simulink model "sampleModel200"  (Simulink 9.1)
settings: Solver=VariableStepAuto  StartTime=0.0  StopTime=10.0  RelTol=1e-3
undefined symbols (not defined in the file): DiscIntNeverNeededParam, magnitude, Newton, Raphson
libraries: simulink x23
settings Model: SuppressorTable="22 serialization::archive 11 0 6 0 0 1 8 0 0 0 0 6 0 0 1 0 22 sampleModel200/cfblk22 0 6 0 0 2 8 0 0 0 0 6 41 Simulink:DataType:WarningOverFlowDetected 0 0 0 6 0  0  0 0 0 0 8 20160608 0 0 0 15 23 17 0 1 40 SimulinkFixedPoint:util:Overflowoccurred 0 0 0  0  8 20160608 0 15 23 17 0 1"  Creator=DELL  LastModifiedBy=DELL
settings DataIOCC: SaveFormat=Dataset
settings OptimizationCC: LifeSpan=auto
settings DebuggingCC: UnderspecifiedInitializationDetection=Simplified  MergeDetectMultiDrivingBlocksExec=error  SFUnexpectedBacktrackingDiag=error  SFNoUnconditionalDefaultTransitionDiag=error  SFExecutionAtInitializationDiag=warning
settings HardwareCC: ProdBitPerPointer=64  ProdBitPerSizeT=64  ProdBitPerPtrDiffT=64  ProdLargestAtomicFloat=Float  ProdIntDivRoundTo=Zero  ProdEndianess=LittleEndian  ProdWordSize=64  ProdHWDeviceType=Intel->x86-64 (Windows64)
settings ModelReferenceCC: PropagateSignalLabelsOutOfModel=on
settings CodeAppCC: StateflowObjectComments=off
settings GRTTargetCC: TargetLangStandard=C99 (ISO)  CombineOutputUpdateFcns=on  GRTInterface=off
settings ConfigComp: CovMetricSettings=dwe  CovHtmlReporting=off  CovSaveCumulativeToWorkspaceVar=off  CovSaveSingleToWorkspaceVar=off  CovExternalEMLEnable=on

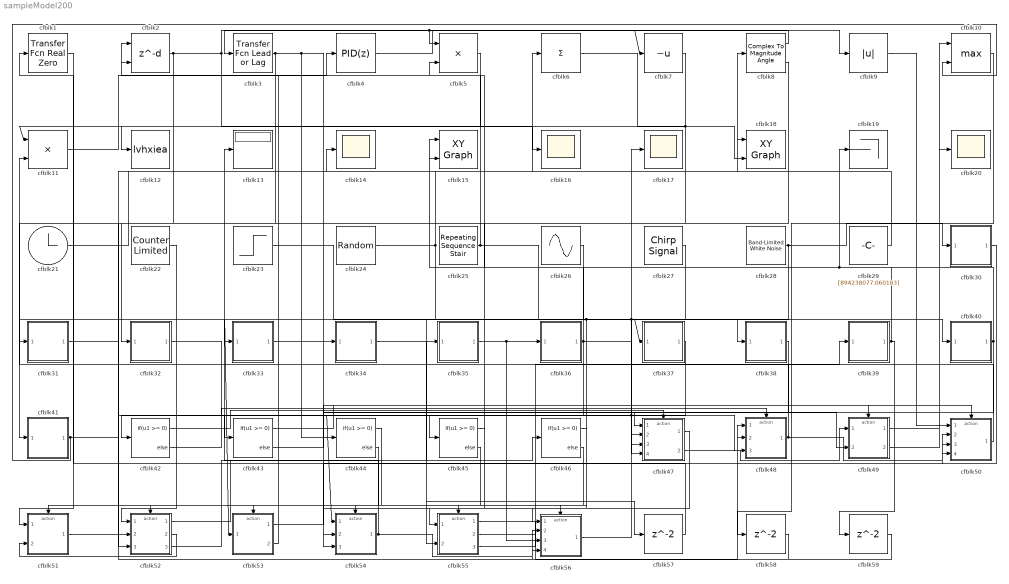
== system sampleModel200 ==
  cfblk1 : simulink/Discrete/Transfer Fcn Real Zero  ZeroZ=0.75  ICPrevInput=0.0  DoSatur=off
      settings: SourceProductName=Simulink  SourceProductBaseCode=SL
  cfblk10 : MinMax  Function=max  Inputs=2
  cfblk11 : Product
  cfblk12 : ToWorkspace  VariableName=lvhxiea  SaveFormat=Timeseries  SampleTime=-1
  cfblk13 : Display
  cfblk{14,16..17,20} (4 alike) : Scope
  cfblk15 : simulink/Sinks/XY Graph  xmin=-1  xmax=1  ymin=-1  ymax=1  st=-1
  cfblk18 : simulink/Sinks/XY Graph  xmin=-1  xmax=1  ymin=-1  ymax=1  st=-1
  cfblk19 : Terminator
  cfblk2 : Delay  DelayLengthSource=Input port  SampleTime=1
      settings: InputPortMap=u0,p1
  cfblk21 : Clock
  cfblk22 : simulink/Sources/Counter Limited  uplimit=[859.000000]  tsamp=-1
  cfblk23 : Step  Time=[38.000000]  Before=[-360941089.850897]  After=[233838912.755649]  SampleTime=0
  cfblk24 : UniformRandomNumber  Minimum=[-6461588901.663700]  Maximum=[4422499536.423707]  Seed=[95995438.000000]  SampleTime=0.1
  cfblk25 : simulink/Sources/Repeating Sequence Stair  OutValues=[-949505601.324327, -713448805.257307]  tsamp=-1  OutMin=[]  OutMax=[]  OutDataTypeStr=double  OutputDataTypeScalingMode=double  OutDataType=fixdt(0,8)  ConRadixGroup=Best Precision: Vector-wise  OutScaling=2^-12
  cfblk26 : Sin  Amplitude=[82135622.117132]  Bias=[-80870349.123243]  SampleTime=0
  cfblk27 : simulink/Sources/Chirp Signal  f1=[749318228.820739]  T=[-649807459.958066]  f2=[-242108775.631314]
  cfblk28 : simulink/Sources/Band-Limited White Noise  Cov=[6378277694.470449]  Ts=0.1  seed=[3428189316.000000]
  cfblk29 : Constant  Value=[894238077.060183]  SampleTime=1
  cfblk3 : simulink/Discrete/Transfer Fcn Lead or Lag  PoleZ=0.95  ZeroZ=0.75  ICPrevOutput=0.0  ICPrevInput=0.0  DoSatur=off
      settings: SourceProductName=Simulink  SourceProductBaseCode=SL
  cfblk30 : Subsystem
  cfblk31 : Subsystem
  cfblk32 : Subsystem
  cfblk33 : Subsystem
  cfblk34 : Subsystem
  cfblk35 : Subsystem
  cfblk36 : Subsystem
  cfblk37 : Subsystem
  cfblk38 : Subsystem
  cfblk39 : Subsystem
  cfblk4 : simulink/Continuous/PID Controller  Controller=PID  TimeDomain=Discrete-time  SampleTime=1  IntegratorMethod=Forward Euler  FilterMethod=Forward Euler  Form=Parallel  UseFilter=on  ControllerParametersSource=internal  P=1  I=1  D=0  N=100  InitialConditionSource=internal  InitialConditionForIntegrator=0  InitialConditionForFilter=0  ExternalReset=none  LimitOutput=off  UpperSaturationLimit=inf  LowerSaturationLimit=-inf  LinearizeAsGain=off  AntiWindupMode=none  Kb=1  TrackingMode=off  Kt=1  PParamMin=[]  PParamMax=[]  IParamMin=[]  IParamMax=[]  DParamMin=[]  DParamMax=[]  NParamMin=[]  NParamMax=[]  KbParamMin=[]  KbParamMax=[]  KtParamMin=[]  KtParamMax=[]  POutMin=[]  POutMax=[]  IOutMin=[]  IOutMax=[]  DOutMin=[]  DOutMax=[]  NOutMin=[]  NOutMax=[]  KbOutMin=[]  KbOutMax=[]  KtOutMin=[]  KtOutMax=[]  IntegratorOutMin=[]  IntegratorOutMax=[]  FilterOutMin=[]  FilterOutMax=[]  SumOutMin=[]  SumOutMax=[]  SumI1OutMin=[]  SumI1OutMax=[]  SumI2OutMin=[]  SumI2OutMax=[]  SumI3OutMin=[]  SumI3OutMax=[]  SumDOutMin=[]  SumDOutMax=[]  SaturationOutMin=[]  SaturationOutMax=[]  IntegratorContinuousStateAttributes=''  IntegratorStateMustResolveToSignalObject=off  IntegratorRTWStateStorageClass=Auto  FilterContinuousStateAttributes=''  FilterStateMustResolveToSignalObject=off  FilterRTWStateStorageClass=Auto  DifferentiatorICPrevScaledInput=0  DifferentiatorOutMin=[]  DifferentiatorOutMax=[]  FilterDiffOutCoefMin=[]  FilterDiffOutCoefMax=[]  SumDenOutMin=[]  SumDenOutMax=[]  SumNumOutMin=[]  SumNumOutMax=[]  ReciprocalOutMin=[]  ReciprocalOutMax=[]  DivideOutMin=[]  DivideOutMax=[]  TunerSelectOption=Transfer Function Based (PID Tuner App)
  cfblk40 : Subsystem
  cfblk41 : Subsystem
  cfblk{42..46} (5 alike) : If  IfExpression=u1 >= 0  SampleTime=1
  cfblk47 : Subsystem  TreatAsAtomicUnit=on
  cfblk48 : Subsystem  TreatAsAtomicUnit=on
  cfblk49 : Subsystem  TreatAsAtomicUnit=on
  cfblk5 : Product  Inputs=**
  cfblk50 : Subsystem  TreatAsAtomicUnit=on
  cfblk51 : Subsystem  TreatAsAtomicUnit=on
  cfblk52 : Subsystem  TreatAsAtomicUnit=on
  cfblk53 : Subsystem  TreatAsAtomicUnit=on
  cfblk54 : Subsystem  TreatAsAtomicUnit=on
  cfblk55 : Subsystem  TreatAsAtomicUnit=on
  cfblk56 : Subsystem  TreatAsAtomicUnit=on
  cfblk57 : Delay  SampleTime=1
  cfblk58 : Delay  SampleTime=1
  cfblk59 : Delay  SampleTime=1
  cfblk6 : Sum  Inputs=+
  cfblk7 : UnaryMinus
  cfblk8 : ComplexToMagnitudeAngle
  cfblk9 : Abs
  wires:
  cfblk7/1 -> cfblk11/1, cfblk55/1(cfblk1)
  cfblk48/1(cfblk2) -> cfblk11/2, cfblk50/4(cfblk12)
  cfblk21/1 -> cfblk8/1
  cfblk39/1(cfblk2) -> cfblk19/1, cfblk5/2, cfblk59/1
  cfblk23/1 -> cfblk37/1(cfblk1), cfblk47/3(cfblk15)
  cfblk9/1 -> cfblk50/1(cfblk1)
  cfblk4/1 -> cfblk9/1
  cfblk56/1(cfblk2) -> cfblk17/1
  cfblk27/1 -> cfblk53/1(cfblk1), cfblk56/1(cfblk1)
  cfblk24/1 -> cfblk6/1, cfblk38/1(cfblk1)
  cfblk8/1 -> cfblk3/1
  cfblk55/1(cfblk2) -> cfblk48/1(cfblk1)
  cfblk5/1 -> cfblk12/1
  cfblk37/1(cfblk2) -> cfblk54/1(cfblk1), cfblk47/2(cfblk14)
  cfblk49/1(cfblk2) -> cfblk10/1
  cfblk36/1(cfblk2) -> cfblk42/1, cfblk40/1(cfblk1), cfblk15/2
  cfblk49/2(cfblk10) -> cfblk20/1
  cfblk22/1 -> cfblk52/1(cfblk1)
  cfblk33/1(cfblk2) -> cfblk34/1(cfblk1)
  cfblk54/1(cfblk2) -> cfblk13/1, cfblk56/2(cfblk12)
  cfblk11/1 -> cfblk4/1
  cfblk50/1(cfblk2) -> cfblk33/1(cfblk1)
  cfblk40/1(cfblk2) -> cfblk15/1, cfblk47/1(cfblk1)
  cfblk35/1(cfblk2) -> cfblk36/1(cfblk1), cfblk56/3(cfblk13)
  cfblk29/1 -> cfblk18/1
  cfblk25/1 -> cfblk2/1, cfblk47/4(cfblk16)
  cfblk51/1(cfblk2) -> cfblk14/1
  cfblk3/1 -> cfblk44/1, cfblk49/2(cfblk9), cfblk32/1(cfblk1)
  cfblk6/1 -> cfblk18/2
  cfblk2/1 -> cfblk5/1, cfblk7/1, cfblk16/1, cfblk52/3(cfblk14)
  cfblk55/2(cfblk13) -> cfblk48/2(cfblk13)
  cfblk30/1(cfblk2) -> cfblk50/2(cfblk10)
  cfblk32/1(cfblk2) -> cfblk45/1
  cfblk8/2 -> cfblk41/1(cfblk1)
  cfblk55/3(cfblk14) -> cfblk39/1(cfblk1)
  cfblk41/1(cfblk2) -> cfblk10/2, cfblk43/1
  cfblk26/1 -> cfblk51/1(cfblk1)
  cfblk47/1(cfblk2) -> cfblk54/2(cfblk11)
  cfblk47/2(cfblk17) -> cfblk49/1(cfblk1)
  cfblk53/1(cfblk2) -> cfblk50/3(cfblk11)
  cfblk31/1(cfblk2) -> cfblk48/3(cfblk14)
  cfblk38/1(cfblk2) -> cfblk54/3(cfblk12)
  cfblk28/1 -> cfblk30/1(cfblk1), cfblk55/2(cfblk12)
  cfblk52/1(cfblk2) -> cfblk35/1(cfblk1)
  cfblk53/2(cfblk7) -> cfblk2/2
  cfblk52/2(cfblk15) -> cfblk51/2(cfblk8)
  cfblk1/1 -> cfblk31/1(cfblk1)
  cfblk52/3(cfblk16) -> cfblk46/1
  cfblk42/1 -> cfblk47/Action
  cfblk42/2 -> cfblk48/Action
  cfblk43/1 -> cfblk49/Action
  cfblk43/2 -> cfblk50/Action
  cfblk44/1 -> cfblk51/Action
  cfblk44/2 -> cfblk52/Action
  cfblk45/1 -> cfblk53/Action
  cfblk45/2 -> cfblk54/Action
  cfblk46/1 -> cfblk55/Action
  cfblk46/2 -> cfblk56/Action
  cfblk34/1(cfblk2) -> cfblk57/1
  cfblk57/1 -> cfblk1/1
  cfblk10/1 -> cfblk58/1
  cfblk58/1 -> cfblk52/2(cfblk13)
  cfblk59/1 -> cfblk56/4(cfblk14)

== system sampleModel200/cfblk30 ==
  cfblk1 : Inport
  cfblk2 : Outport
  wires:
  cfblk1/1 -> cfblk2/1

== system sampleModel200/cfblk31 ==
  cfblk1 : Inport
  cfblk2 : Outport
  wires:
  cfblk1/1 -> cfblk2/1

== system sampleModel200/cfblk32 ==
  cfblk1 : Inport
  cfblk2 : Outport
  wires:
  cfblk1/1 -> cfblk2/1

== system sampleModel200/cfblk33 ==
  cfblk1 : Inport
  cfblk2 : Outport
  wires:
  cfblk1/1 -> cfblk2/1

== system sampleModel200/cfblk34 ==
  cfblk1 : Inport
  cfblk2 : Outport
  wires:
  cfblk1/1 -> cfblk2/1

== system sampleModel200/cfblk35 ==
  cfblk1 : Inport
  cfblk2 : Outport
  wires:
  cfblk1/1 -> cfblk2/1

== system sampleModel200/cfblk36 ==
  cfblk1 : Inport
  cfblk2 : Outport
  wires:
  cfblk1/1 -> cfblk2/1

== system sampleModel200/cfblk37 ==
  cfblk1 : Inport
  cfblk2 : Outport
  wires:
  cfblk1/1 -> cfblk2/1

== system sampleModel200/cfblk38 ==
  cfblk1 : Inport
  cfblk2 : Outport
  wires:
  cfblk1/1 -> cfblk2/1

== system sampleModel200/cfblk39 ==
  cfblk1 : Inport
  cfblk2 : Outport
  wires:
  cfblk1/1 -> cfblk2/1

== system sampleModel200/cfblk40 ==
  cfblk1 : Inport
  cfblk2 : Outport
  wires:
  cfblk1/1 -> cfblk2/1

== system sampleModel200/cfblk41 ==
  cfblk1 : Inport
  cfblk2 : Outport
  wires:
  cfblk1/1 -> cfblk2/1

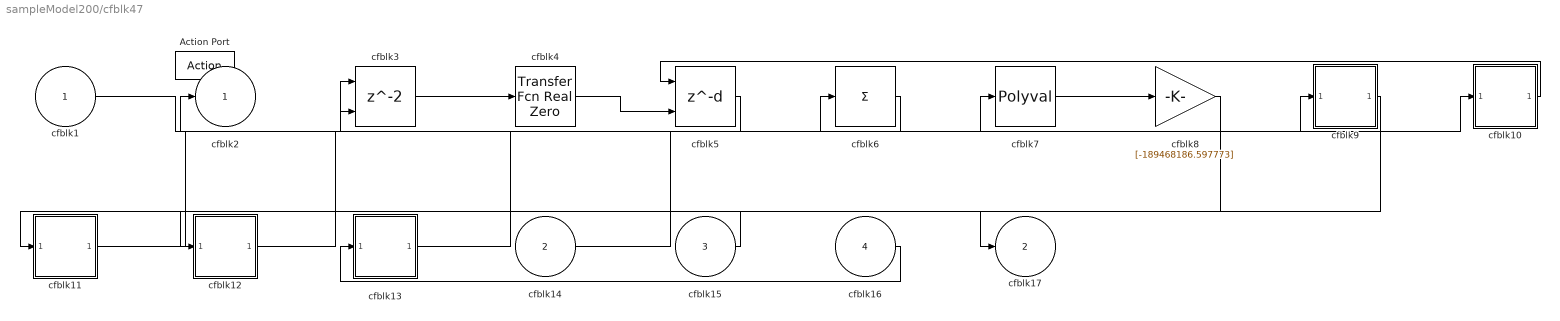
== system sampleModel200/cfblk47 ==
  cfblk1 : Inport
  cfblk14 : Inport  Port=2
  cfblk15 : Inport  Port=3
  cfblk16 : Inport  Port=4
  Action Port : ActionPort  ActionType=then
  cfblk10 : Subsystem
  cfblk11 : Subsystem
  cfblk12 : Subsystem
  cfblk13 : Subsystem
  cfblk3 : Delay  ShowEnablePort=on
      settings: InputPortMap=u0,e6
  cfblk4 : simulink/Discrete/Transfer Fcn Real Zero  ZeroZ=0.75  ICPrevInput=0.0  DoSatur=off
      settings: SourceProductName=Simulink  SourceProductBaseCode=SL
  cfblk5 : Delay  DelayLengthSource=Input port
      settings: InputPortMap=u0,p1
  cfblk6 : Sum  Inputs=+
  cfblk7 : Polyval  Coefs=[ +2.081618890e-019, -1.441693666e-014, +4.719686976e-010, -8.536869453e-006, +1.621573104e-001, -8.087801117e+001 ]
  cfblk8 : Gain  Gain=[-189468186.597773]
  cfblk9 : Subsystem
  cfblk2 : Outport
  cfblk17 : Outport  Port=2
  wires:
  cfblk7/1 -> cfblk8/1
  cfblk13/1(cfblk2) -> cfblk10/1(cfblk1)
  cfblk3/1 -> cfblk4/1
  cfblk16/1 -> cfblk13/1(cfblk1)
  cfblk14/1 -> cfblk7/1
  cfblk10/1(cfblk2) -> cfblk5/1
  cfblk11/1(cfblk2) -> cfblk3/1
  cfblk5/1 -> cfblk2/1
  cfblk4/1 -> cfblk5/2
  cfblk12/1(cfblk2) -> cfblk9/1(cfblk1)
  cfblk9/1(cfblk2) -> cfblk17/1
  cfblk15/1 -> cfblk12/1(cfblk1)
  cfblk8/1 -> cfblk11/1(cfblk1)
  cfblk6/1 -> cfblk3/2
  cfblk1/1 -> cfblk6/1

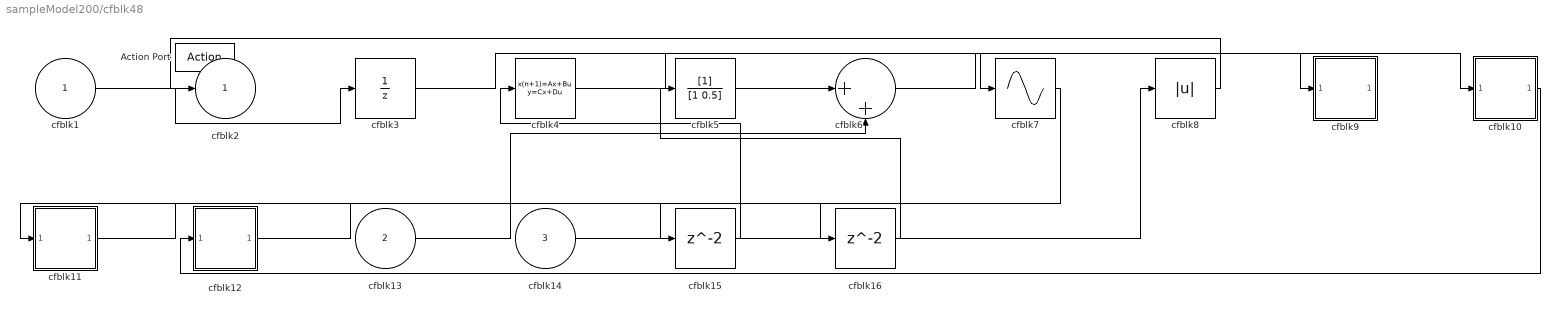
== system sampleModel200/cfblk48 ==
  cfblk1 : Inport
  cfblk13 : Inport  Port=2
  cfblk14 : Inport  Port=3
  Action Port : ActionPort  ActionType=else
  cfblk10 : Subsystem
  cfblk11 : Subsystem
  cfblk12 : Subsystem
  cfblk15 : Delay
  cfblk16 : Delay
  cfblk3 : UnitDelay  SampleTime=-1
  cfblk4 : DiscreteStateSpace  SampleTime=-1
  cfblk5 : DiscreteFilter
  cfblk6 : Sum  Inputs=|++
  cfblk7 : Sin  TimeSource=Use external signal  SampleTime=0
  cfblk8 : Abs
  cfblk9 : Subsystem
  cfblk2 : Outport
  wires:
  cfblk4/1 -> cfblk7/1
  cfblk7/1 -> cfblk11/1(cfblk1)
  cfblk14/1 -> cfblk8/1
  cfblk10/1(cfblk2) -> cfblk12/1(cfblk1)
  cfblk5/1 -> cfblk6/1
  cfblk8/1 -> cfblk2/1
  cfblk13/1 -> cfblk6/2
  cfblk3/1 -> cfblk9/1(cfblk1)
  cfblk6/1 -> cfblk10/1(cfblk1)
  cfblk1/1 -> cfblk3/1
  cfblk11/1(cfblk2) -> cfblk15/1
  cfblk15/1 -> cfblk4/1
  cfblk12/1(cfblk2) -> cfblk16/1
  cfblk16/1 -> cfblk5/1

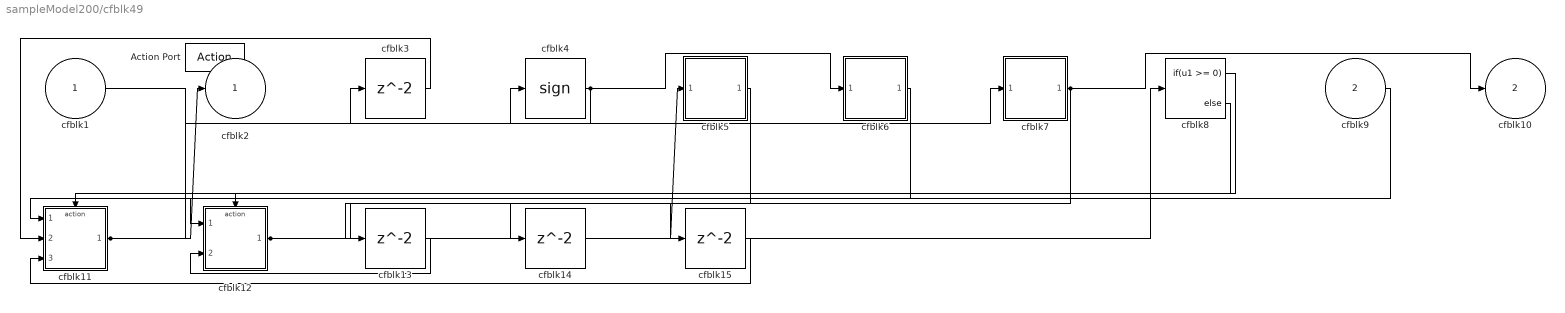
== system sampleModel200/cfblk49 ==
  cfblk1 : Inport
  cfblk9 : Inport  Port=2
  Action Port : ActionPort  ActionType=then
  cfblk11 : Subsystem  TreatAsAtomicUnit=on
  cfblk12 : Subsystem  TreatAsAtomicUnit=on
  cfblk{3,13..15} (4 alike) : Delay
  cfblk4 : Signum
  cfblk5 : Subsystem
  cfblk6 : Subsystem
  cfblk7 : Subsystem
  cfblk8 : If  IfExpression=u1 >= 0  SampleTime=1
  cfblk2 : Outport
  cfblk10 : Outport  Port=2
  wires:
  cfblk9/1 -> cfblk11/1(cfblk1)
  cfblk11/1(cfblk2) -> cfblk2/1, cfblk7/1(cfblk1)
  cfblk6/1(cfblk2) -> cfblk12/1(cfblk1)
  cfblk7/1(cfblk2) -> cfblk10/1, cfblk13/1
  cfblk3/1 -> cfblk11/2(cfblk12)
  cfblk4/1 -> cfblk3/1, cfblk6/1(cfblk1)
  cfblk1/1 -> cfblk4/1
  cfblk12/1(cfblk2) -> cfblk5/1(cfblk1), cfblk15/1
  cfblk8/1 -> cfblk11/Action
  cfblk8/2 -> cfblk12/Action
  cfblk13/1 -> cfblk12/2(cfblk15)
  cfblk5/1(cfblk2) -> cfblk14/1
  cfblk14/1 -> cfblk8/1
  cfblk15/1 -> cfblk11/3(cfblk13)

== system sampleModel200/cfblk50 ==
  cfblk1 : Inport
  cfblk10 : Inport  Port=2
  cfblk11 : Inport  Port=3
  cfblk12 : Inport  Port=4
  Action Port : ActionPort  ActionType=else
  cfblk13 : Delay
  cfblk3 : Rounding
  cfblk4 : Abs
  cfblk5 : Subsystem
  cfblk6 : Subsystem
  cfblk7 : Subsystem
  cfblk8 : Subsystem
  cfblk9 : Subsystem
  cfblk2 : Outport
  wires:
  cfblk4/1 -> cfblk9/1(cfblk1)
  cfblk5/1(cfblk2) -> cfblk7/1(cfblk1)
  cfblk9/1(cfblk2) -> cfblk2/1
  cfblk1/1 -> cfblk6/1(cfblk1)
  cfblk10/1 -> cfblk8/1(cfblk1)
  cfblk11/1 -> cfblk4/1
  cfblk8/1(cfblk2) -> cfblk3/1
  cfblk7/1(cfblk2) -> cfblk13/1
  cfblk13/1 -> cfblk5/1(cfblk1)

== system sampleModel200/cfblk51 ==
  cfblk1 : Inport
  cfblk8 : Inport  Port=2
  Action Port : ActionPort  ActionType=then
  cfblk3 : DiscreteIntegrator  SampleTime=-1  ICPrevOutput=DiscIntNeverNeededParam  ICPrevScaledInput=DiscIntNeverNeededParam
  cfblk4 : MinMax  Function=max  Inputs=3
  cfblk5 : Subsystem
  cfblk6 : Subsystem
  cfblk7 : Subsystem
  cfblk9 : Delay
  cfblk2 : Outport
  wires:
  cfblk3/1 -> cfblk6/1(cfblk1)
  cfblk5/1(cfblk2) -> cfblk4/1, cfblk7/1(cfblk1)
  cfblk6/1(cfblk2) -> cfblk4/2
  cfblk1/1 -> cfblk2/1
  cfblk7/1(cfblk2) -> cfblk4/3
  cfblk8/1 -> cfblk5/1(cfblk1)
  cfblk4/1 -> cfblk9/1
  cfblk9/1 -> cfblk3/1

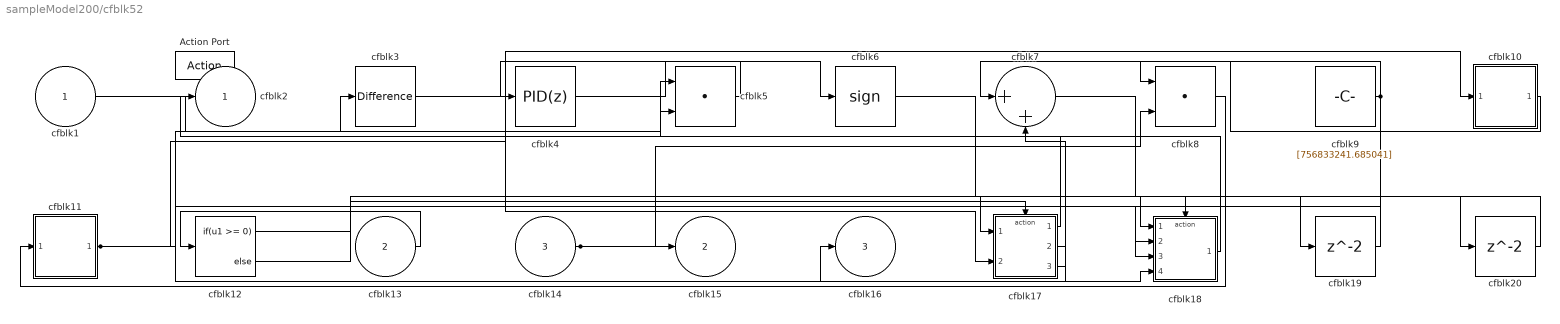
== system sampleModel200/cfblk52 ==
  cfblk1 : Inport
  cfblk13 : Inport  Port=2
  cfblk14 : Inport  Port=3
  Action Port : ActionPort  ActionType=else
  cfblk10 : Subsystem
  cfblk11 : Subsystem
  cfblk12 : If  IfExpression=u1 >= 0  SampleTime=1
  cfblk17 : Subsystem  TreatAsAtomicUnit=on
  cfblk18 : Subsystem  TreatAsAtomicUnit=on
  cfblk19 : Delay
  cfblk20 : Delay
  cfblk3 : simulink/Discrete/Difference  ICPrevInput=0.0  OutMin=[]  OutMax=[]  OutDataTypeStr=Inherit: Inherit via back propagation  OutDataType=fixdt(1, 16)  OutScaling=2^-10  DoSatur=off
  cfblk4 : simulink/Continuous/PID Controller  Controller=PID  TimeDomain=Discrete-time  SampleTime=-1  IntegratorMethod=Forward Euler  FilterMethod=Forward Euler  Form=Parallel  UseFilter=on  ControllerParametersSource=internal  P=1  I=1  D=0  N=100  InitialConditionSource=internal  InitialConditionForIntegrator=0  InitialConditionForFilter=0  ExternalReset=none  LimitOutput=off  UpperSaturationLimit=inf  LowerSaturationLimit=-inf  LinearizeAsGain=off  AntiWindupMode=none  Kb=1  TrackingMode=off  Kt=1  PParamMin=[]  PParamMax=[]  IParamMin=[]  IParamMax=[]  DParamMin=[]  DParamMax=[]  NParamMin=[]  NParamMax=[]  KbParamMin=[]  KbParamMax=[]  KtParamMin=[]  KtParamMax=[]  POutMin=[]  POutMax=[]  IOutMin=[]  IOutMax=[]  DOutMin=[]  DOutMax=[]  NOutMin=[]  NOutMax=[]  KbOutMin=[]  KbOutMax=[]  KtOutMin=[]  KtOutMax=[]  IntegratorOutMin=[]  IntegratorOutMax=[]  FilterOutMin=[]  FilterOutMax=[]  SumOutMin=[]  SumOutMax=[]  SumI1OutMin=[]  SumI1OutMax=[]  SumI2OutMin=[]  SumI2OutMax=[]  SumI3OutMin=[]  SumI3OutMax=[]  SumDOutMin=[]  SumDOutMax=[]  SaturationOutMin=[]  SaturationOutMax=[]  IntegratorContinuousStateAttributes=''  IntegratorStateMustResolveToSignalObject=off  IntegratorRTWStateStorageClass=Auto  FilterContinuousStateAttributes=''  FilterStateMustResolveToSignalObject=off  FilterRTWStateStorageClass=Auto  DifferentiatorICPrevScaledInput=0  DifferentiatorOutMin=[]  DifferentiatorOutMax=[]  FilterDiffOutCoefMin=[]  FilterDiffOutCoefMax=[]  SumDenOutMin=[]  SumDenOutMax=[]  SumNumOutMin=[]  SumNumOutMax=[]  ReciprocalOutMin=[]  ReciprocalOutMax=[]  DivideOutMin=[]  DivideOutMax=[]  TunerSelectOption=Transfer Function Based (PID Tuner App)
  cfblk5 : DotProduct  InputSameDT=on  OutDataTypeStr=Inherit: Inherit via internal rule
  cfblk6 : Signum
  cfblk7 : Sum  Inputs=|++
  cfblk8 : DotProduct  InputSameDT=on  OutDataTypeStr=Inherit: Inherit via internal rule
  cfblk9 : Constant  Value=[756833241.685041]  SampleTime=1
  cfblk2 : Outport
  cfblk15 : Outport  Port=2
  cfblk16 : Outport  Port=3
  wires:
  cfblk4/1 -> cfblk6/1
  cfblk14/1 -> cfblk15/1, cfblk8/2
  cfblk8/1 -> cfblk11/1(cfblk1)
  cfblk13/1 -> cfblk12/1
  cfblk1/1 -> cfblk3/1
  cfblk17/1(cfblk2) -> cfblk5/1
  cfblk11/1(cfblk2) -> cfblk10/1(cfblk1), cfblk5/2, cfblk18/2(cfblk10), cfblk18/4(cfblk12)
  cfblk3/1 -> cfblk17/2(cfblk10)
  cfblk5/1 -> cfblk4/1
  cfblk17/2(cfblk11) -> cfblk16/1
  cfblk18/1(cfblk2) -> cfblk2/1
  cfblk10/1(cfblk2) -> cfblk7/1
  cfblk9/1 -> cfblk8/1, cfblk18/3(cfblk11)
  cfblk17/3(cfblk12) -> cfblk7/2
  cfblk12/1 -> cfblk17/Action
  cfblk12/2 -> cfblk18/Action
  cfblk6/1 -> cfblk19/1
  cfblk19/1 -> cfblk18/1(cfblk1)
  cfblk7/1 -> cfblk20/1
  cfblk20/1 -> cfblk17/1(cfblk1)

== system sampleModel200/cfblk53 ==
  cfblk1 : Inport
  Action Port : ActionPort  ActionType=then
  cfblk3 : Constant  Value=[-39529075.697824]  SampleTime=1
  cfblk4 : Subsystem
  cfblk5 : Subsystem
  cfblk6 : Subsystem
  cfblk2 : Outport
  cfblk7 : Outport  Port=2
  wires:
  cfblk5/1(cfblk2) -> cfblk6/1(cfblk1)
  cfblk4/1(cfblk2) -> cfblk5/1(cfblk1)
  cfblk1/1 -> cfblk4/1(cfblk1)
  cfblk3/1 -> cfblk7/1
  cfblk6/1(cfblk2) -> cfblk2/1

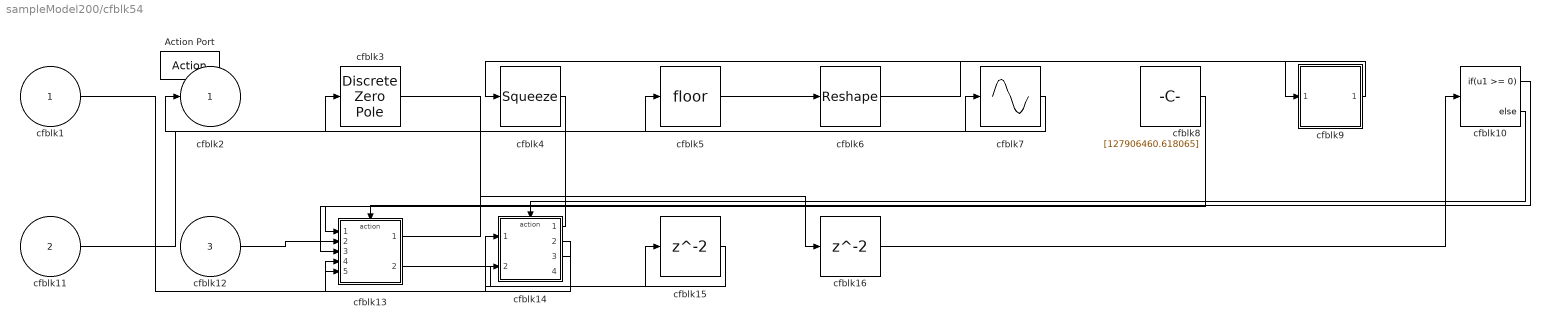
== system sampleModel200/cfblk54 ==
  cfblk1 : Inport
  cfblk11 : Inport  Port=2
  cfblk12 : Inport  Port=3
  Action Port : ActionPort  ActionType=else
  cfblk10 : If  IfExpression=u1 >= 0  SampleTime=1
  cfblk13 : Subsystem  TreatAsAtomicUnit=on
  cfblk14 : Subsystem  TreatAsAtomicUnit=on
  cfblk15 : Delay
  cfblk16 : Delay
  cfblk3 : DiscreteZeroPole  Poles=[0 0.5]  Gain=1  SampleTime=-1
  cfblk4 : Squeeze
  cfblk5 : Rounding
  cfblk6 : Reshape
  cfblk7 : Sin  TimeSource=Use external signal  SampleTime=0
  cfblk8 : Constant  Value=[127906460.618065]  SampleTime=1
  cfblk9 : Subsystem
  cfblk2 : Outport
  wires:
  cfblk7/1 -> cfblk2/1
  cfblk9/1(cfblk2) -> cfblk4/1
  cfblk8/1 -> cfblk13/1(cfblk1)
  cfblk12/1 -> cfblk13/2(cfblk11)
  cfblk1/1 -> cfblk14/1(cfblk1)
  cfblk11/1 -> cfblk5/1
  cfblk14/1(cfblk2) -> cfblk3/1
  cfblk13/1(cfblk2) -> cfblk7/1
  cfblk5/1 -> cfblk6/1
  cfblk4/1 -> cfblk13/3(cfblk12)
  cfblk6/1 -> cfblk9/1(cfblk1)
  cfblk14/2(cfblk15) -> cfblk13/4(cfblk13)
  cfblk14/3(cfblk16) -> cfblk13/5(cfblk14)
  cfblk10/1 -> cfblk13/Action
  cfblk10/2 -> cfblk14/Action
  cfblk13/2(cfblk15) -> cfblk15/1
  cfblk15/1 -> cfblk14/2(cfblk14)
  cfblk3/1 -> cfblk16/1
  cfblk16/1 -> cfblk10/1

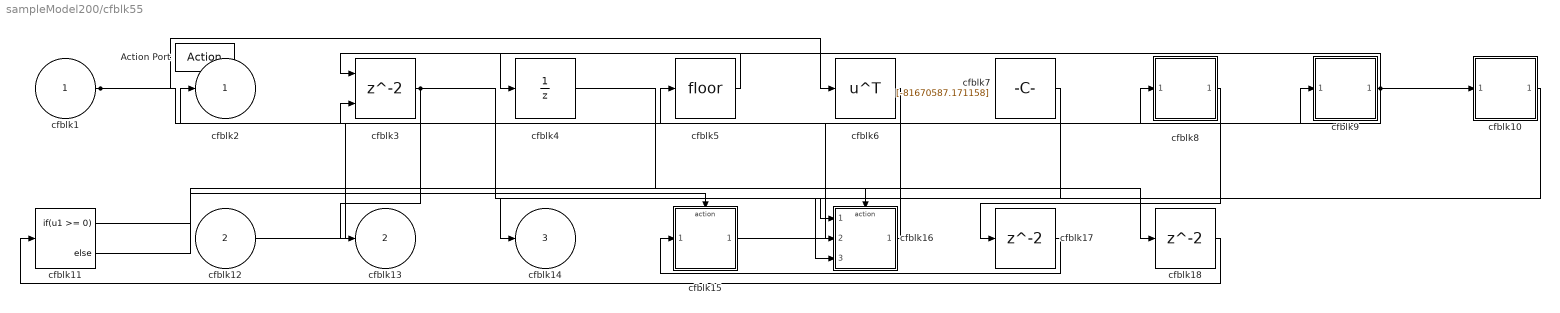
== system sampleModel200/cfblk55 ==
  cfblk1 : Inport
  cfblk12 : Inport  Port=2
  Action Port : ActionPort  ActionType=then
  cfblk10 : Subsystem
  cfblk11 : If  IfExpression=u1 >= 0  SampleTime=1
  cfblk15 : Subsystem  TreatAsAtomicUnit=on
  cfblk16 : Subsystem  TreatAsAtomicUnit=on
  cfblk17 : Delay
  cfblk18 : Delay
  cfblk3 : Delay  ShowEnablePort=on
      settings: InputPortMap=u0,e6
  cfblk4 : UnitDelay  SampleTime=-1
  cfblk5 : Rounding
  cfblk6 : Math  Operator=transpose  SaturateOnIntegerOverflow=on
  cfblk7 : Constant  Value=[-81670587.171158]  SampleTime=1
  cfblk8 : Subsystem
  cfblk9 : Subsystem
  cfblk2 : Outport
  cfblk13 : Outport  Port=2
  cfblk14 : Outport  Port=3
  wires:
  cfblk12/1 -> cfblk9/1(cfblk1)
  cfblk3/1 -> cfblk13/1, cfblk16/3(cfblk10)
  cfblk15/1(cfblk2) -> cfblk8/1(cfblk1)
  cfblk1/1 -> cfblk6/1, cfblk3/2
  cfblk5/1 -> cfblk4/1
  cfblk9/1(cfblk2) -> cfblk2/1, cfblk10/1(cfblk1), cfblk3/1
  cfblk16/1(cfblk2) -> cfblk5/1
  cfblk10/1(cfblk2) -> cfblk16/1(cfblk1)
  cfblk7/1 -> cfblk14/1
  cfblk6/1 -> cfblk16/2(cfblk9)
  cfblk11/1 -> cfblk15/Action
  cfblk11/2 -> cfblk16/Action
  cfblk8/1(cfblk2) -> cfblk17/1
  cfblk17/1 -> cfblk15/1(cfblk1)
  cfblk4/1 -> cfblk18/1
  cfblk18/1 -> cfblk11/1

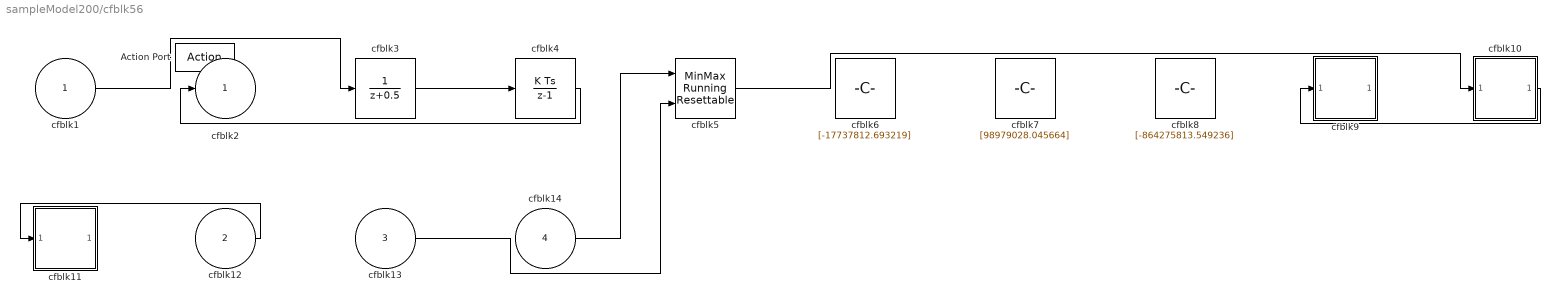
== system sampleModel200/cfblk56 ==
  cfblk1 : Inport
  cfblk12 : Inport  Port=2
  cfblk13 : Inport  Port=3
  cfblk14 : Inport  Port=4
  Action Port : ActionPort  ActionType=else
  cfblk10 : Subsystem
  cfblk11 : Subsystem
  cfblk3 : DiscreteTransferFcn
  cfblk4 : DiscreteIntegrator  SampleTime=-1  ICPrevOutput=DiscIntNeverNeededParam  ICPrevScaledInput=DiscIntNeverNeededParam
  cfblk5 : simulink/Math Operations/MinMax Running Resettable  Function=min  vinit=0.0
  cfblk6 : Constant  Value=[-17737812.693219]  SampleTime=1
  cfblk7 : Constant  Value=[98979028.045664]  SampleTime=1
  cfblk8 : Constant  Value=[-864275813.549236]  SampleTime=1
  cfblk9 : Subsystem
  cfblk2 : Outport
  wires:
  cfblk5/1 -> cfblk10/1(cfblk1)
  cfblk4/1 -> cfblk2/1
  cfblk10/1(cfblk2) -> cfblk9/1(cfblk1)
  cfblk12/1 -> cfblk11/1(cfblk1)
  cfblk3/1 -> cfblk4/1
  cfblk1/1 -> cfblk3/1
  cfblk14/1 -> cfblk5/1
  cfblk13/1 -> cfblk5/2

== system sampleModel200/cfblk47/cfblk10 ==
  cfblk1 : Inport
  cfblk2 : Outport
  wires:
  cfblk1/1 -> cfblk2/1

== system sampleModel200/cfblk47/cfblk11 ==
  cfblk1 : Inport
  cfblk2 : Outport
  wires:
  cfblk1/1 -> cfblk2/1

== system sampleModel200/cfblk47/cfblk12 ==
  cfblk1 : Inport
  cfblk2 : Outport
  wires:
  cfblk1/1 -> cfblk2/1

== system sampleModel200/cfblk47/cfblk13 ==
  cfblk1 : Inport
  cfblk2 : Outport
  wires:
  cfblk1/1 -> cfblk2/1

== system sampleModel200/cfblk47/cfblk9 ==
  cfblk1 : Inport
  cfblk2 : Outport
  wires:
  cfblk1/1 -> cfblk2/1

== system sampleModel200/cfblk48/cfblk10 ==
  cfblk1 : Inport
  cfblk2 : Outport
  wires:
  cfblk1/1 -> cfblk2/1

== system sampleModel200/cfblk48/cfblk11 ==
  cfblk1 : Inport
  cfblk2 : Outport
  wires:
  cfblk1/1 -> cfblk2/1

== system sampleModel200/cfblk48/cfblk12 ==
  cfblk1 : Inport
  cfblk2 : Outport
  wires:
  cfblk1/1 -> cfblk2/1

== system sampleModel200/cfblk48/cfblk9 ==
  cfblk1 : Inport
  cfblk2 : Outport
  wires:
  cfblk1/1 -> cfblk2/1

== system sampleModel200/cfblk49/cfblk11 ==
  cfblk1 : Inport
  cfblk12 : Inport  Port=2
  cfblk13 : Inport  Port=3
  Action Port : ActionPort  ActionType=then
  cfblk10 : Subsystem
  cfblk11 : Subsystem
  cfblk14 : Delay
  cfblk3 : UnitDelay  SampleTime=-1
  cfblk4 : simulink/Discrete/Transfer Fcn Lead or Lag  PoleZ=0.95  ZeroZ=0.75  ICPrevOutput=0.0  ICPrevInput=0.0  DoSatur=off
      settings: SourceProductName=Simulink  SourceProductBaseCode=SL
  cfblk5 : simulink/Math Operations/Slider Gain  gain=1  low=0  high=2
  cfblk6 : simulink/Math Operations/Slider Gain  gain=1  low=0  high=2
  cfblk7 : ComplexToMagnitudeAngle
  cfblk8 : Constant  Value=[-606562205.070100]  SampleTime=1
  cfblk9 : Subsystem
  cfblk2 : Outport
  wires:
  cfblk7/1 -> cfblk10/1(cfblk1)
  cfblk3/1 -> cfblk7/1
  cfblk5/1 -> cfblk6/1
  cfblk10/1(cfblk2) -> cfblk9/1(cfblk1)
  cfblk13/1 -> cfblk11/1(cfblk1)
  cfblk11/1(cfblk2) -> cfblk5/1
  cfblk6/1 -> cfblk4/1
  cfblk12/1 -> cfblk2/1
  cfblk7/2 -> cfblk14/1
  cfblk14/1 -> cfblk3/1

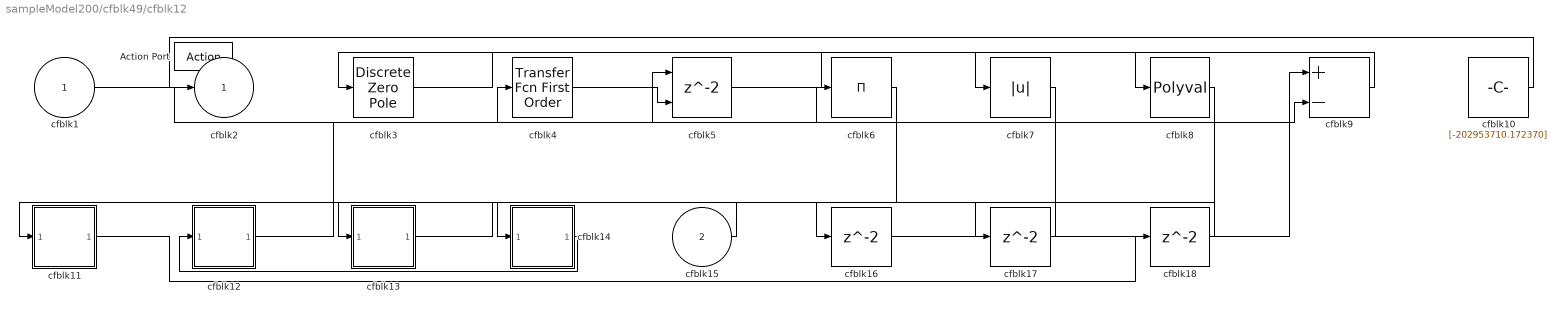
== system sampleModel200/cfblk49/cfblk12 ==
  cfblk1 : Inport
  cfblk15 : Inport  Port=2
  Action Port : ActionPort  ActionType=else
  cfblk10 : Constant  Value=[-202953710.172370]  SampleTime=1
  cfblk11 : Subsystem
  cfblk12 : Subsystem
  cfblk13 : Subsystem
  cfblk14 : Subsystem
  cfblk16 : Delay
  cfblk17 : Delay
  cfblk18 : Delay
  cfblk3 : DiscreteZeroPole  Poles=[0 0.5]  Gain=1  SampleTime=-1
  cfblk4 : simulink/Discrete/Transfer Fcn First Order  PoleZ=0.95  ICPrevOutput=0.0  DoSatur=off
      settings: SourceProductName=Simulink
  cfblk5 : Delay  ShowEnablePort=on
      settings: InputPortMap=u0,e6
  cfblk6 : Product  Inputs=*
  cfblk7 : Abs
  cfblk8 : Polyval  Coefs=[ +2.081618890e-019, -1.441693666e-014, +4.719686976e-010, -8.536869453e-006, +1.621573104e-001, -8.087801117e+001 ]
  cfblk9 : Sum  Inputs=+-
  cfblk2 : Outport
  wires:
  cfblk6/1 -> cfblk11/1(cfblk1)
  cfblk9/1 -> cfblk3/1
  cfblk14/1(cfblk2) -> cfblk12/1(cfblk1)
  cfblk7/1 -> cfblk13/1(cfblk1)
  cfblk10/1 -> cfblk2/1
  cfblk5/1 -> cfblk7/1
  cfblk12/1(cfblk2) -> cfblk4/1
  cfblk15/1 -> cfblk14/1(cfblk1)
  cfblk3/1 -> cfblk8/1
  cfblk4/1 -> cfblk5/2
  cfblk1/1 -> cfblk9/2
  cfblk8/1 -> cfblk16/1
  cfblk16/1 -> cfblk9/1
  cfblk13/1(cfblk2) -> cfblk17/1
  cfblk17/1 -> cfblk5/1
  cfblk11/1(cfblk2) -> cfblk18/1
  cfblk18/1 -> cfblk6/1

== system sampleModel200/cfblk49/cfblk5 ==
  cfblk1 : Inport
  cfblk2 : Outport
  wires:
  cfblk1/1 -> cfblk2/1

== system sampleModel200/cfblk49/cfblk6 ==
  cfblk1 : Inport
  cfblk2 : Outport
  wires:
  cfblk1/1 -> cfblk2/1

== system sampleModel200/cfblk49/cfblk7 ==
  cfblk1 : Inport
  cfblk2 : Outport
  wires:
  cfblk1/1 -> cfblk2/1

== system sampleModel200/cfblk50/cfblk5 ==
  cfblk1 : Inport
  cfblk2 : Outport
  wires:
  cfblk1/1 -> cfblk2/1

== system sampleModel200/cfblk50/cfblk6 ==
  cfblk1 : Inport
  cfblk2 : Outport
  wires:
  cfblk1/1 -> cfblk2/1

== system sampleModel200/cfblk50/cfblk7 ==
  cfblk1 : Inport
  cfblk2 : Outport
  wires:
  cfblk1/1 -> cfblk2/1

== system sampleModel200/cfblk50/cfblk8 ==
  cfblk1 : Inport
  cfblk2 : Outport
  wires:
  cfblk1/1 -> cfblk2/1

== system sampleModel200/cfblk50/cfblk9 ==
  cfblk1 : Inport
  cfblk2 : Outport
  wires:
  cfblk1/1 -> cfblk2/1

== system sampleModel200/cfblk51/cfblk5 ==
  cfblk1 : Inport
  cfblk2 : Outport
  wires:
  cfblk1/1 -> cfblk2/1

== system sampleModel200/cfblk51/cfblk6 ==
  cfblk1 : Inport
  cfblk2 : Outport
  wires:
  cfblk1/1 -> cfblk2/1

== system sampleModel200/cfblk51/cfblk7 ==
  cfblk1 : Inport
  cfblk2 : Outport
  wires:
  cfblk1/1 -> cfblk2/1

== system sampleModel200/cfblk52/cfblk10 ==
  cfblk1 : Inport
  cfblk2 : Outport
  wires:
  cfblk1/1 -> cfblk2/1

== system sampleModel200/cfblk52/cfblk11 ==
  cfblk1 : Inport
  cfblk2 : Outport
  wires:
  cfblk1/1 -> cfblk2/1

== system sampleModel200/cfblk52/cfblk17 ==
  cfblk1 : Inport
  cfblk10 : Inport  Port=2
  Action Port : ActionPort  ActionType=then
  cfblk13 : Delay
  cfblk3 : Signum
  cfblk4 : simulink/Math Operations/MinMax Running Resettable  Function=min  vinit=0.0
  cfblk5 : Constant  Value=[-921191467.517140]  SampleTime=1
  cfblk6 : Subsystem
  cfblk7 : Subsystem
  cfblk8 : Subsystem
  cfblk9 : Subsystem
  cfblk2 : Outport
  cfblk11 : Outport  Port=2
  cfblk12 : Outport  Port=3
  wires:
  cfblk9/1(cfblk2) -> cfblk2/1
  cfblk1/1 -> cfblk3/1
  cfblk8/1(cfblk2) -> cfblk7/1(cfblk1)
  cfblk10/1 -> cfblk8/1(cfblk1)
  cfblk7/1(cfblk2) -> cfblk9/1(cfblk1)
  cfblk5/1 -> cfblk12/1
  cfblk3/1 -> cfblk4/2
  cfblk4/1 -> cfblk11/1, cfblk6/1(cfblk1)
  cfblk6/1(cfblk2) -> cfblk13/1
  cfblk13/1 -> cfblk4/1

== system sampleModel200/cfblk52/cfblk18 ==
  cfblk1 : Inport
  cfblk10 : Inport  Port=2
  cfblk11 : Inport  Port=3
  cfblk12 : Inport  Port=4
  Action Port : ActionPort  ActionType=else
  cfblk3 : Delay
  cfblk4 : Sqrt  SaturateOnIntegerOverflow=on
  cfblk5 : Product
  cfblk6 : Sum  Inputs=+-
  cfblk7 : Subsystem
  cfblk8 : Subsystem
  cfblk9 : Subsystem
  cfblk2 : Outport
  wires:
  cfblk7/1(cfblk2) -> cfblk8/1(cfblk1)
  cfblk9/1(cfblk2) -> cfblk5/1
  cfblk5/1 -> cfblk2/1
  cfblk10/1 -> cfblk6/1
  cfblk1/1 -> cfblk4/1
  cfblk4/1 -> cfblk7/1(cfblk1)
  cfblk8/1(cfblk2) -> cfblk5/2
  cfblk12/1 -> cfblk3/1
  cfblk11/1 -> cfblk6/2
  cfblk3/1 -> cfblk9/1(cfblk1)

== system sampleModel200/cfblk53/cfblk4 ==
  cfblk1 : Inport
  cfblk2 : Outport
  wires:
  cfblk1/1 -> cfblk2/1

== system sampleModel200/cfblk53/cfblk5 ==
  cfblk1 : Inport
  cfblk2 : Outport
  wires:
  cfblk1/1 -> cfblk2/1

== system sampleModel200/cfblk53/cfblk6 ==
  cfblk1 : Inport
  cfblk2 : Outport
  wires:
  cfblk1/1 -> cfblk2/1

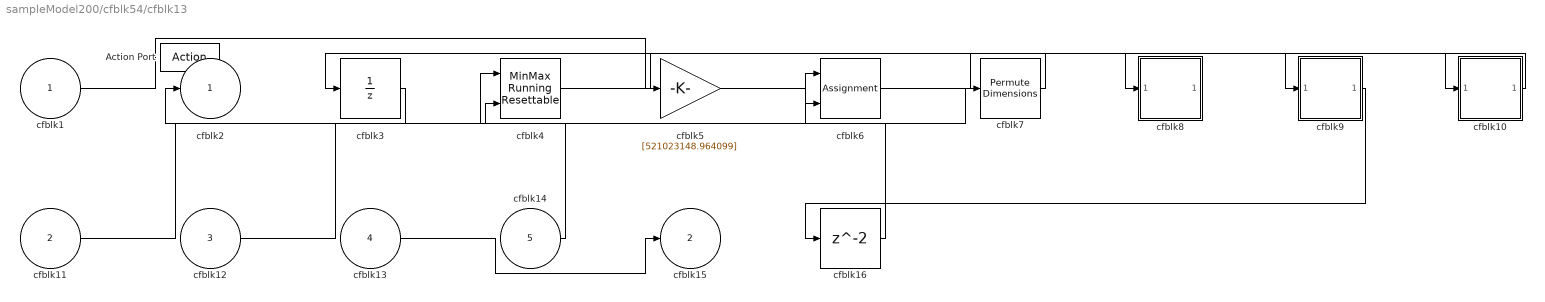
== system sampleModel200/cfblk54/cfblk13 ==
  cfblk1 : Inport
  cfblk11 : Inport  Port=2
  cfblk12 : Inport  Port=3
  cfblk13 : Inport  Port=4
  cfblk14 : Inport  Port=5
  Action Port : ActionPort  ActionType=then
  cfblk10 : Subsystem
  cfblk16 : Delay
  cfblk3 : UnitDelay  SampleTime=-1
  cfblk4 : simulink/Math Operations/MinMax Running Resettable  Function=min  vinit=0.0
  cfblk5 : Gain  Gain=[521023148.964099]
  cfblk6 : Assignment  DiagnosticForDimensions=Warning  IndexOptions=Index vector (dialog)  Indices=1  OutputSizes=1
  cfblk7 : PermuteDimensions
  cfblk8 : Subsystem
  cfblk9 : Subsystem
  cfblk2 : Outport
  cfblk15 : Outport  Port=2
  wires:
  cfblk4/1 -> cfblk10/1(cfblk1)
  cfblk10/1(cfblk2) -> cfblk9/1(cfblk1)
  cfblk14/1 -> cfblk4/2
  cfblk1/1 -> cfblk5/1
  cfblk3/1 -> cfblk2/1
  cfblk13/1 -> cfblk15/1
  cfblk7/1 -> cfblk3/1
  cfblk6/1 -> cfblk8/1(cfblk1)
  cfblk12/1 -> cfblk6/1
  cfblk11/1 -> cfblk7/1
  cfblk5/1 -> cfblk6/2
  cfblk9/1(cfblk2) -> cfblk16/1
  cfblk16/1 -> cfblk4/1

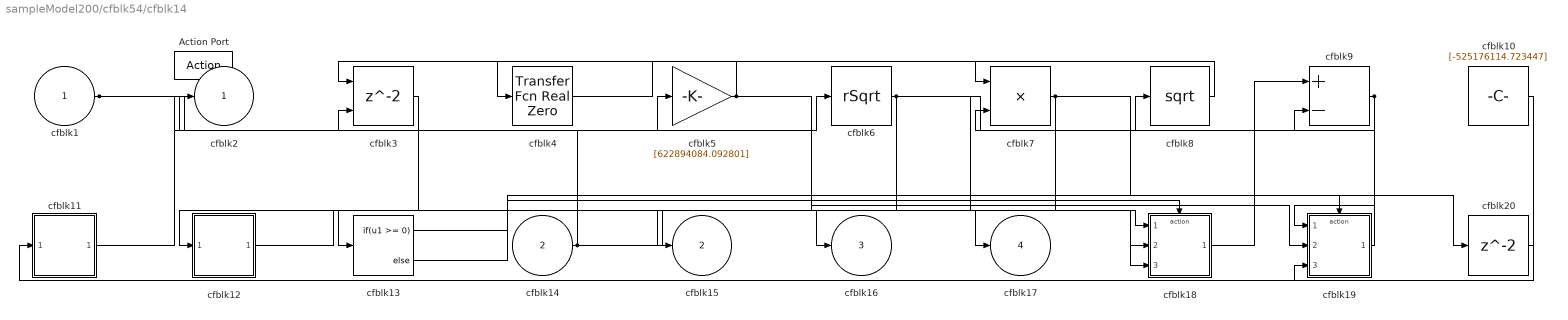
== system sampleModel200/cfblk54/cfblk14 ==
  cfblk1 : Inport
  cfblk14 : Inport  Port=2
  Action Port : ActionPort  ActionType=else
  cfblk10 : Constant  Value=[-525176114.723447]  SampleTime=1
  cfblk11 : Subsystem
  cfblk12 : Subsystem
  cfblk13 : If  IfExpression=u1 >= 0  SampleTime=1
  cfblk18 : Subsystem  TreatAsAtomicUnit=on
  cfblk19 : Subsystem  TreatAsAtomicUnit=on
  cfblk20 : Delay
  cfblk3 : Delay  ShowEnablePort=on
      settings: InputPortMap=u0,e6
  cfblk4 : simulink/Discrete/Transfer Fcn Real Zero  ZeroZ=0.75  ICPrevInput=0.0  DoSatur=off
      settings: SourceProductName=Simulink  SourceProductBaseCode=SL
  cfblk5 : Gain  Gain=[622894084.092801]
  cfblk6 : Sqrt  Operator=rSqrt  AlgorithmType=Newton-Raphson  SaturateOnIntegerOverflow=on
  cfblk7 : Product
  cfblk8 : Sqrt  SaturateOnIntegerOverflow=on
  cfblk9 : Sum  Inputs=+-
  cfblk2 : Outport
  cfblk15 : Outport  Port=2
  cfblk16 : Outport  Port=3
  cfblk17 : Outport  Port=4
  wires:
  cfblk8/1 -> cfblk4/1
  cfblk7/1 -> cfblk12/1(cfblk1), cfblk20/1
  cfblk10/1 -> cfblk11/1(cfblk1)
  cfblk18/1(cfblk2) -> cfblk9/1
  cfblk1/1 -> cfblk6/1, cfblk3/2
  cfblk11/1(cfblk2) -> cfblk5/1
  cfblk14/1 -> cfblk16/1, cfblk2/1
  cfblk5/1 -> cfblk3/1, cfblk19/2(cfblk14), cfblk18/2(cfblk13)
  cfblk3/1 -> cfblk13/1
  cfblk4/1 -> cfblk7/1
  cfblk6/1 -> cfblk9/2, cfblk15/1, cfblk18/1(cfblk1), cfblk18/3(cfblk14)
  cfblk19/1(cfblk2) -> cfblk8/1
  cfblk9/1 -> cfblk19/1(cfblk1), cfblk7/2
  cfblk12/1(cfblk2) -> cfblk17/1
  cfblk13/1 -> cfblk18/Action
  cfblk13/2 -> cfblk19/Action
  cfblk20/1 -> cfblk19/3(cfblk15)

== system sampleModel200/cfblk54/cfblk9 ==
  cfblk1 : Inport
  cfblk2 : Outport
  wires:
  cfblk1/1 -> cfblk2/1

== system sampleModel200/cfblk55/cfblk10 ==
  cfblk1 : Inport
  cfblk2 : Outport
  wires:
  cfblk1/1 -> cfblk2/1

== system sampleModel200/cfblk55/cfblk15 ==
  cfblk1 : Inport
  Action Port : ActionPort  ActionType=then
  cfblk10 : Delay
  cfblk3 : simulink/Discrete/Transfer Fcn First Order  PoleZ=0.95  ICPrevOutput=0.0  DoSatur=off
      settings: SourceProductName=Simulink
  cfblk4 : Abs
  cfblk5 : Gain  Gain=[-962958558.003246]
  cfblk6 : Subsystem
  cfblk7 : Subsystem
  cfblk8 : Subsystem
  cfblk9 : Delay
  cfblk2 : Outport
  wires:
  cfblk3/1 -> cfblk7/1(cfblk1)
  cfblk7/1(cfblk2) -> cfblk8/1(cfblk1)
  cfblk5/1 -> cfblk6/1(cfblk1)
  cfblk1/1 -> cfblk2/1
  cfblk8/1(cfblk2) -> cfblk4/1
  cfblk4/1 -> cfblk9/1
  cfblk9/1 -> cfblk3/1
  cfblk6/1(cfblk2) -> cfblk10/1
  cfblk10/1 -> cfblk5/1

== system sampleModel200/cfblk55/cfblk16 ==
  cfblk1 : Inport
  cfblk9 : Inport  Port=2
  cfblk10 : Inport  Port=3
  Action Port : ActionPort  ActionType=else
  cfblk3 : simulink/Continuous/PID Controller (2DOF)  Controller=PID  TimeDomain=Discrete-time  SampleTime=-1  IntegratorMethod=Forward Euler  FilterMethod=Forward Euler  Form=Parallel  UseFilter=on  ControllerParametersSource=internal  P=1  I=1  D=0  N=100  b=1  c=1  InitialConditionSource=internal  InitialConditionForIntegrator=0  InitialConditionForFilter=0  ExternalReset=none  LimitOutput=off  UpperSaturationLimit=inf  LowerSaturationLimit=-inf  LinearizeAsGain=off  AntiWindupMode=none  Kb=1  TrackingMode=off  Kt=1  PParamMin=[]  PParamMax=[]  IParamMin=[]  IParamMax=[]  DParamMin=[]  DParamMax=[]  NParamMin=[]  NParamMax=[]  bParamMin=[]  bParamMax=[]  cParamMin=[]  cParamMax=[]  KbParamMin=[]  KbParamMax=[]  KtParamMin=[]  KtParamMax=[]  POutMin=[]  POutMax=[]  IOutMin=[]  IOutMax=[]  DOutMin=[]  DOutMax=[]  NOutMin=[]  NOutMax=[]  bOutMin=[]  bOutMax=[]  cOutMin=[]  cOutMax=[]  KbOutMin=[]  KbOutMax=[]  KtOutMin=[]  KtOutMax=[]  IntegratorOutMin=[]  IntegratorOutMax=[]  FilterOutMin=[]  FilterOutMax=[]  SumOutMin=[]  SumOutMax=[]  Sum1OutMin=[]  Sum1OutMax=[]  Sum2OutMin=[]  Sum2OutMax=[]  Sum3OutMin=[]  Sum3OutMax=[]  SumI1OutMin=[]  SumI1OutMax=[]  SumI2OutMin=[]  SumI2OutMax=[]  SumI3OutMin=[]  SumI3OutMax=[]  SumDOutMin=[]  SumDOutMax=[]  SaturationOutMin=[]  SaturationOutMax=[]  IntegratorContinuousStateAttributes=''  IntegratorStateMustResolveToSignalObject=off  IntegratorRTWStateStorageClass=Auto  FilterContinuousStateAttributes=''  FilterStateMustResolveToSignalObject=off  FilterRTWStateStorageClass=Auto  DifferentiatorICPrevScaledInput=0  DifferentiatorOutMin=[]  DifferentiatorOutMax=[]  FilterDiffOutCoefMin=[]  FilterDiffOutCoefMax=[]  SumDenOutMin=[]  SumDenOutMax=[]  SumNumOutMin=[]  SumNumOutMax=[]  ReciprocalOutMin=[]  ReciprocalOutMax=[]  DivideOutMin=[]  DivideOutMax=[]  TunerSelectOption=Transfer Function Based (PID Tuner App)
  cfblk4 : DiscreteStateSpace  SampleTime=-1
  cfblk5 : DiscreteZeroPole  Poles=[0 0.5]  Gain=1  SampleTime=-1
  cfblk6 : DotProduct  InputSameDT=on  OutDataTypeStr=Inherit: Inherit via internal rule
  cfblk7 : Subsystem
  cfblk8 : Subsystem
  cfblk2 : Outport
  wires:
  cfblk9/1 -> cfblk8/1(cfblk1)
  cfblk1/1 -> cfblk3/1, cfblk6/2
  cfblk4/1 -> cfblk5/1
  cfblk3/1 -> cfblk7/1(cfblk1)
  cfblk5/1 -> cfblk6/1
  cfblk7/1(cfblk2) -> cfblk4/1
  cfblk8/1(cfblk2) -> cfblk2/1
  cfblk10/1 -> cfblk3/2

== system sampleModel200/cfblk55/cfblk8 ==
  cfblk1 : Inport
  cfblk2 : Outport
  wires:
  cfblk1/1 -> cfblk2/1

== system sampleModel200/cfblk55/cfblk9 ==
  cfblk1 : Inport
  cfblk2 : Outport
  wires:
  cfblk1/1 -> cfblk2/1

== system sampleModel200/cfblk56/cfblk10 ==
  cfblk1 : Inport
  cfblk2 : Outport
  wires:
  cfblk1/1 -> cfblk2/1

== system sampleModel200/cfblk56/cfblk11 ==
  cfblk1 : Inport
  cfblk2 : Outport
  wires:
  cfblk1/1 -> cfblk2/1

== system sampleModel200/cfblk56/cfblk9 ==
  cfblk1 : Inport
  cfblk2 : Outport
  wires:
  cfblk1/1 -> cfblk2/1

== system sampleModel200/cfblk49/cfblk11/cfblk10 ==
  cfblk1 : Inport
  cfblk2 : Outport
  wires:
  cfblk1/1 -> cfblk2/1

== system sampleModel200/cfblk49/cfblk11/cfblk11 ==
  cfblk1 : Inport
  cfblk2 : Outport
  wires:
  cfblk1/1 -> cfblk2/1

== system sampleModel200/cfblk49/cfblk11/cfblk9 ==
  cfblk1 : Inport
  cfblk2 : Outport
  wires:
  cfblk1/1 -> cfblk2/1

== system sampleModel200/cfblk49/cfblk12/cfblk11 ==
  cfblk1 : Inport
  cfblk2 : Outport
  wires:
  cfblk1/1 -> cfblk2/1

== system sampleModel200/cfblk49/cfblk12/cfblk12 ==
  cfblk1 : Inport
  cfblk2 : Outport
  wires:
  cfblk1/1 -> cfblk2/1

== system sampleModel200/cfblk49/cfblk12/cfblk13 ==
  cfblk1 : Inport
  cfblk2 : Outport
  wires:
  cfblk1/1 -> cfblk2/1

== system sampleModel200/cfblk49/cfblk12/cfblk14 ==
  cfblk1 : Inport
  cfblk2 : Outport
  wires:
  cfblk1/1 -> cfblk2/1

== system sampleModel200/cfblk52/cfblk17/cfblk6 ==
  cfblk1 : Inport
  cfblk2 : Outport
  wires:
  cfblk1/1 -> cfblk2/1

== system sampleModel200/cfblk52/cfblk17/cfblk7 ==
  cfblk1 : Inport
  cfblk2 : Outport
  wires:
  cfblk1/1 -> cfblk2/1

== system sampleModel200/cfblk52/cfblk17/cfblk8 ==
  cfblk1 : Inport
  cfblk2 : Outport
  wires:
  cfblk1/1 -> cfblk2/1

== system sampleModel200/cfblk52/cfblk17/cfblk9 ==
  cfblk1 : Inport
  cfblk2 : Outport
  wires:
  cfblk1/1 -> cfblk2/1

== system sampleModel200/cfblk52/cfblk18/cfblk7 ==
  cfblk1 : Inport
  cfblk2 : Outport
  wires:
  cfblk1/1 -> cfblk2/1

== system sampleModel200/cfblk52/cfblk18/cfblk8 ==
  cfblk1 : Inport
  cfblk2 : Outport
  wires:
  cfblk1/1 -> cfblk2/1

== system sampleModel200/cfblk52/cfblk18/cfblk9 ==
  cfblk1 : Inport
  cfblk2 : Outport
  wires:
  cfblk1/1 -> cfblk2/1

== system sampleModel200/cfblk54/cfblk13/cfblk10 ==
  cfblk1 : Inport
  cfblk2 : Outport
  wires:
  cfblk1/1 -> cfblk2/1

== system sampleModel200/cfblk54/cfblk13/cfblk8 ==
  cfblk1 : Inport
  cfblk2 : Outport
  wires:
  cfblk1/1 -> cfblk2/1

== system sampleModel200/cfblk54/cfblk13/cfblk9 ==
  cfblk1 : Inport
  cfblk2 : Outport
  wires:
  cfblk1/1 -> cfblk2/1

== system sampleModel200/cfblk54/cfblk14/cfblk11 ==
  cfblk1 : Inport
  cfblk2 : Outport
  wires:
  cfblk1/1 -> cfblk2/1

== system sampleModel200/cfblk54/cfblk14/cfblk12 ==
  cfblk1 : Inport
  cfblk2 : Outport
  wires:
  cfblk1/1 -> cfblk2/1

== system sampleModel200/cfblk54/cfblk14/cfblk18 ==
  cfblk1 : Inport
  cfblk13 : Inport  Port=2
  cfblk14 : Inport  Port=3
  Action Port : ActionPort  ActionType=then
  cfblk10 : Subsystem
  cfblk11 : Subsystem
  cfblk12 : Subsystem
  cfblk3 : Math  Operator=magnitude^2  SaturateOnIntegerOverflow=on
  cfblk4 : Reshape
  cfblk5 : Product
  cfblk6 : Constant  Value=[-145163053.332344]  SampleTime=1
  cfblk7 : Subsystem
  cfblk8 : Subsystem
  cfblk9 : Subsystem
  cfblk2 : Outport
  wires:
  cfblk3/1 -> cfblk5/1
  cfblk6/1 -> cfblk7/1(cfblk1)
  cfblk5/1 -> cfblk2/1
  cfblk14/1 -> cfblk11/1(cfblk1)
  cfblk7/1(cfblk2) -> cfblk8/1(cfblk1)
  cfblk9/1(cfblk2) -> cfblk5/2
  cfblk8/1(cfblk2) -> cfblk3/1
  cfblk12/1(cfblk2) -> cfblk9/1(cfblk1)
  cfblk4/1 -> cfblk10/1(cfblk1)
  cfblk13/1 -> cfblk12/1(cfblk1)
  cfblk11/1(cfblk2) -> cfblk4/1

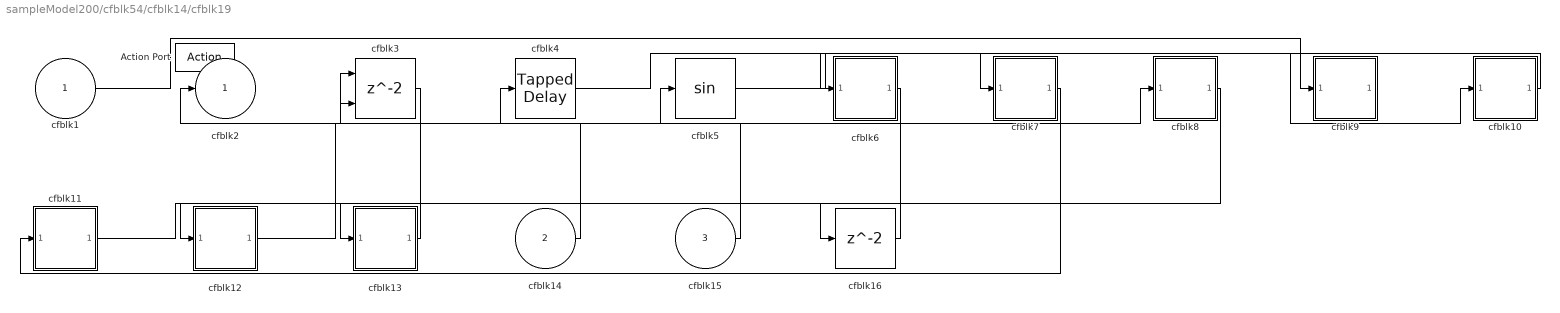
== system sampleModel200/cfblk54/cfblk14/cfblk19 ==
  cfblk1 : Inport
  cfblk14 : Inport  Port=2
  cfblk15 : Inport  Port=3
  Action Port : ActionPort  ActionType=else
  cfblk10 : Subsystem
  cfblk11 : Subsystem
  cfblk12 : Subsystem
  cfblk13 : Subsystem
  cfblk16 : Delay
  cfblk3 : Delay  ShowEnablePort=on
      settings: InputPortMap=u0,e6
  cfblk4 : simulink/Discrete/Tapped Delay  vinit=0.0  samptime=-1  NumDelays=1  DelayOrder=Oldest  includeCurrent=off
  cfblk5 : Trigonometry
  cfblk6 : Subsystem
  cfblk7 : Subsystem
  cfblk8 : Subsystem
  cfblk9 : Subsystem
  cfblk2 : Outport
  wires:
  cfblk1/1 -> cfblk9/1(cfblk1)
  cfblk4/1 -> cfblk10/1(cfblk1)
  cfblk13/1(cfblk2) -> cfblk2/1
  cfblk7/1(cfblk2) -> cfblk11/1(cfblk1)
  cfblk8/1(cfblk2) -> cfblk13/1(cfblk1)
  cfblk15/1 -> cfblk4/1
  cfblk12/1(cfblk2) -> cfblk8/1(cfblk1)
  cfblk5/1 -> cfblk7/1(cfblk1)
  cfblk14/1 -> cfblk3/1
  cfblk6/1(cfblk2) -> cfblk3/2
  cfblk10/1(cfblk2) -> cfblk6/1(cfblk1)
  cfblk3/1 -> cfblk12/1(cfblk1)
  cfblk11/1(cfblk2) -> cfblk16/1
  cfblk16/1 -> cfblk5/1

== system sampleModel200/cfblk55/cfblk15/cfblk6 ==
  cfblk1 : Inport
  cfblk2 : Outport
  wires:
  cfblk1/1 -> cfblk2/1

== system sampleModel200/cfblk55/cfblk15/cfblk7 ==
  cfblk1 : Inport
  cfblk2 : Outport
  wires:
  cfblk1/1 -> cfblk2/1

== system sampleModel200/cfblk55/cfblk15/cfblk8 ==
  cfblk1 : Inport
  cfblk2 : Outport
  wires:
  cfblk1/1 -> cfblk2/1

== system sampleModel200/cfblk55/cfblk16/cfblk7 ==
  cfblk1 : Inport
  cfblk2 : Outport
  wires:
  cfblk1/1 -> cfblk2/1

== system sampleModel200/cfblk55/cfblk16/cfblk8 ==
  cfblk1 : Inport
  cfblk2 : Outport
  wires:
  cfblk1/1 -> cfblk2/1

== system sampleModel200/cfblk54/cfblk14/cfblk18/cfblk10 ==
  cfblk1 : Inport
  cfblk2 : Outport
  wires:
  cfblk1/1 -> cfblk2/1

== system sampleModel200/cfblk54/cfblk14/cfblk18/cfblk11 ==
  cfblk1 : Inport
  cfblk2 : Outport
  wires:
  cfblk1/1 -> cfblk2/1

== system sampleModel200/cfblk54/cfblk14/cfblk18/cfblk12 ==
  cfblk1 : Inport
  cfblk2 : Outport
  wires:
  cfblk1/1 -> cfblk2/1

== system sampleModel200/cfblk54/cfblk14/cfblk18/cfblk7 ==
  cfblk1 : Inport
  cfblk2 : Outport
  wires:
  cfblk1/1 -> cfblk2/1

== system sampleModel200/cfblk54/cfblk14/cfblk18/cfblk8 ==
  cfblk1 : Inport
  cfblk2 : Outport
  wires:
  cfblk1/1 -> cfblk2/1

== system sampleModel200/cfblk54/cfblk14/cfblk18/cfblk9 ==
  cfblk1 : Inport
  cfblk2 : Outport
  wires:
  cfblk1/1 -> cfblk2/1

== system sampleModel200/cfblk54/cfblk14/cfblk19/cfblk10 ==
  cfblk1 : Inport
  cfblk2 : Outport
  wires:
  cfblk1/1 -> cfblk2/1

== system sampleModel200/cfblk54/cfblk14/cfblk19/cfblk11 ==
  cfblk1 : Inport
  cfblk2 : Outport
  wires:
  cfblk1/1 -> cfblk2/1

== system sampleModel200/cfblk54/cfblk14/cfblk19/cfblk12 ==
  cfblk1 : Inport
  cfblk2 : Outport
  wires:
  cfblk1/1 -> cfblk2/1

== system sampleModel200/cfblk54/cfblk14/cfblk19/cfblk13 ==
  cfblk1 : Inport
  cfblk2 : Outport
  wires:
  cfblk1/1 -> cfblk2/1

== system sampleModel200/cfblk54/cfblk14/cfblk19/cfblk6 ==
  cfblk1 : Inport
  cfblk2 : Outport
  wires:
  cfblk1/1 -> cfblk2/1

== system sampleModel200/cfblk54/cfblk14/cfblk19/cfblk7 ==
  cfblk1 : Inport
  cfblk2 : Outport
  wires:
  cfblk1/1 -> cfblk2/1

== system sampleModel200/cfblk54/cfblk14/cfblk19/cfblk8 ==
  cfblk1 : Inport
  cfblk2 : Outport
  wires:
  cfblk1/1 -> cfblk2/1

== system sampleModel200/cfblk54/cfblk14/cfblk19/cfblk9 ==
  cfblk1 : Inport
  cfblk2 : Outport
  wires:
  cfblk1/1 -> cfblk2/1
